simulink model "modelPredictiveControl_v0"  (R2024b)
settings: Solver=FixedStepAuto  StartTime=0.0  StopTime=80  FixedStep=0.01  RelTol=1e-3
undefined symbols (not defined in the file or in its folder): C, del_t, initial_conditions
libraries: mpclib x3
(part 1 of 2)
settings Model: Creator=sagar  LastModifiedBy=Sakar
settings RTWCC: GPUComputeCapability=3.5

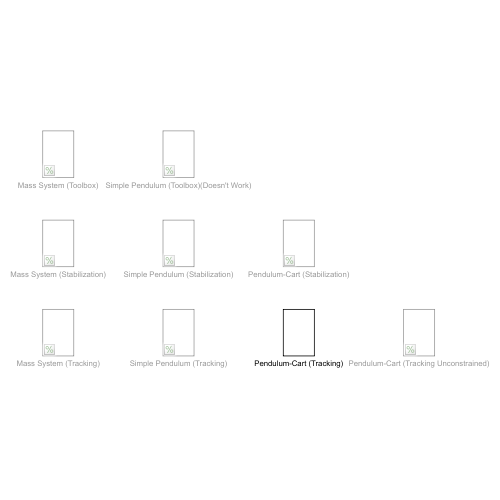
[thumbnail: Simulink's stored preview of the top-level diagram]
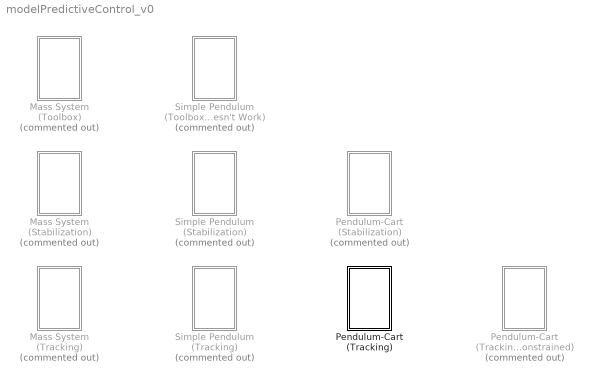
== system modelPredictiveControl_v0 ==
  Mass System (Stabilization) : Subsystem  Commented=on
  Mass System (Toolbox) : Subsystem  Commented=on
  Mass System (Tracking) : Subsystem  Commented=on
  Pendulum-Cart (Stabilization) : Subsystem  Commented=on
  Pendulum-Cart (Tracking Unconstrained) : Subsystem  Commented=on
  Pendulum-Cart (Tracking) : Subsystem
  Simple Pendulum (Stabilization) : Subsystem  Commented=on
  Simple Pendulum (Toolbox)(Doesn't Work) : Subsystem  Commented=on
  Simple Pendulum (Tracking) : Subsystem  Commented=on

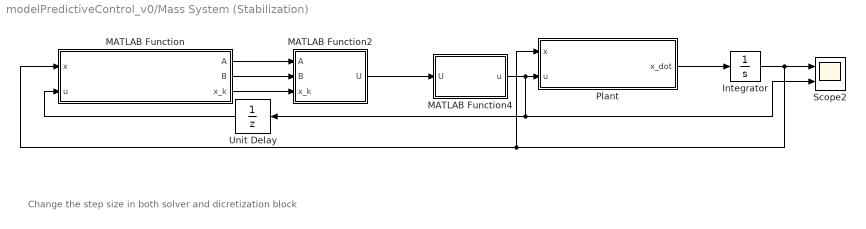
== system modelPredictiveControl_v0/Mass System (Stabilization) ==
  note: Change the step size in both solver and dicretization block
  Integrator : Integrator  InitialCondition=initial_conditions
  MATLAB Function : MATLAB Function  TreatAsAtomicUnit=on
  MATLAB Function2 : MATLAB Function  TreatAsAtomicUnit=on
  MATLAB Function4 : MATLAB Function  TreatAsAtomicUnit=on
  Plant : MATLAB Function  TreatAsAtomicUnit=on
  Scope2 : Scope  NumInputPorts=2
  Unit Delay : UnitDelay  SampleTime=-1  HasFrameUpgradeWarning=on
  wires:
  Plant/1(x_dot) -> Integrator/1
  Integrator/1 -> Scope2/1, Plant/1(x), MATLAB Function/1(x)
  MATLAB Function2/1(U) -> MATLAB Function4/1(U)
  MATLAB Function/1(A) -> MATLAB Function2/1(A)
  MATLAB Function/2(B) -> MATLAB Function2/2(B)
  MATLAB Function/3(x_k) -> MATLAB Function2/3(x_k)
  MATLAB Function4/1(u) -> Scope2/2, Unit Delay/1, Plant/2(u)
  Unit Delay/1 -> MATLAB Function/2(u)

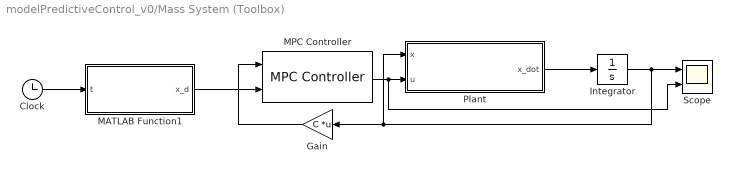
== system modelPredictiveControl_v0/Mass System (Toolbox) ==
  Clock : Clock
  Gain : Gain  Gain=C  Multiplication=Matrix(K*u)
  Integrator : Integrator  InitialCondition=initial_conditions
  MATLAB Function1 : MATLAB Function  TreatAsAtomicUnit=on
  MPC Controller : mpclib/MPC Controller  SCDEnableBlockLinearizationSpecification=on  mpcobj=mpc1  is_multiple=0  enable_value=0  return_u0=off  updateMPCinCallerWorkspace=on  md_inport=off  mv_inport=off  uref_inport=off  return_cost=off  return_mvseq=off  return_qpstatus=off  return_xseq=off  return_state=off  return_ovseq=off  state_inport=off  umin_inport=off  umax_inport=off  ymin_inport=off  ymax_inport=off  cc_inport=off  ywt_inport=off  uwt_inport=off  duwt_inport=off  rhoeps_inport=off  pm_inport=off  MaximumP=10  HorizonChoice=FixedHorizon  n_ts=0.01  n_p=50  n_mv=1  n_md=0  n_ud=0  n_mo=1  n_uo=0  BlockDataType=double  SampleTimeInherited=off  switch_inport=off
  Plant : MATLAB Function  TreatAsAtomicUnit=on
  Scope : Scope  NumInputPorts=2
  wires:
  MPC Controller/1 -> Scope/2, Plant/2(u)
  Plant/1(x_dot) -> Integrator/1
  Integrator/1 -> Scope/1, Plant/1(x), Gain/1
  Clock/1 -> MATLAB Function1/1(t)
  MATLAB Function1/1(x_d) -> MPC Controller/2
  Gain/1 -> MPC Controller/1

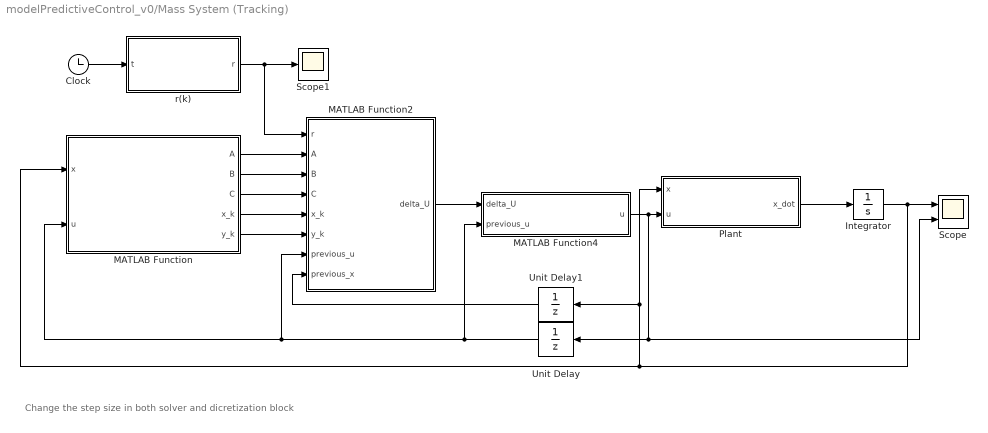
== system modelPredictiveControl_v0/Mass System (Tracking) ==
  note: Change the step size in both solver and dicretization block
  Clock : Clock
  Integrator : Integrator  InitialCondition=initial_conditions
  MATLAB Function : MATLAB Function  TreatAsAtomicUnit=on
  MATLAB Function2 : MATLAB Function  TreatAsAtomicUnit=on
  MATLAB Function4 : MATLAB Function  TreatAsAtomicUnit=on
  Plant : MATLAB Function  TreatAsAtomicUnit=on
  Scope : Scope  NumInputPorts=2
  Scope1 : Scope
  Unit Delay : UnitDelay  SampleTime=-1  HasFrameUpgradeWarning=on
  Unit Delay1 : UnitDelay  SampleTime=-1  HasFrameUpgradeWarning=on
  r(k) : MATLAB Function  TreatAsAtomicUnit=on
  wires:
  Plant/1(x_dot) -> Integrator/1
  Integrator/1 -> Scope/1, Unit Delay1/1, Plant/1(x), MATLAB Function/1(x)
  MATLAB Function2/1(delta_U) -> MATLAB Function4/1(delta_U)
  MATLAB Function/1(A) -> MATLAB Function2/2(A)
  MATLAB Function/2(B) -> MATLAB Function2/3(B)
  MATLAB Function/4(x_k) -> MATLAB Function2/5(x_k)
  MATLAB Function4/1(u) -> Unit Delay/1, Scope/2, Plant/2(u)
  Unit Delay/1 -> MATLAB Function4/2(previous_u), MATLAB Function/2(u), MATLAB Function2/7(previous_u)
  Clock/1 -> r(k)/1(t)
  r(k)/1(r) -> MATLAB Function2/1(r), Scope1/1
  MATLAB Function/3(C) -> MATLAB Function2/4(C)
  Unit Delay1/1 -> MATLAB Function2/8(previous_x)
  MATLAB Function/5(y_k) -> MATLAB Function2/6(y_k)

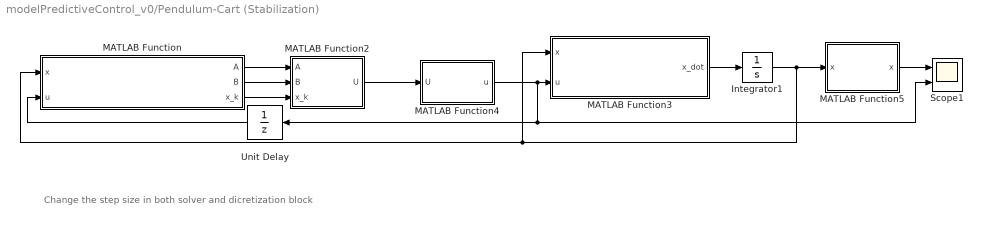
== system modelPredictiveControl_v0/Pendulum-Cart (Stabilization) ==
  note: Change the step size in both solver and dicretization block
  Integrator1 : Integrator  InitialCondition=initial_conditions
  MATLAB Function : MATLAB Function  TreatAsAtomicUnit=on
  MATLAB Function2 : MATLAB Function  TreatAsAtomicUnit=on
  MATLAB Function3 : MATLAB Function  TreatAsAtomicUnit=on
  MATLAB Function4 : MATLAB Function  TreatAsAtomicUnit=on
  MATLAB Function5 : MATLAB Function  TreatAsAtomicUnit=on
  Scope1 : Scope  NumInputPorts=2
  Unit Delay : UnitDelay  SampleTime=-1  HasFrameUpgradeWarning=on
  wires:
  MATLAB Function4/1(u) -> MATLAB Function3/2(u), Unit Delay/1, Scope1/2
  Unit Delay/1 -> MATLAB Function/2(u)
  MATLAB Function2/1(U) -> MATLAB Function4/1(U)
  MATLAB Function/3(x_k) -> MATLAB Function2/3(x_k)
  MATLAB Function/1(A) -> MATLAB Function2/1(A)
  Integrator1/1 -> MATLAB Function5/1("x "), MATLAB Function3/1(x), MATLAB Function/1(x)
  MATLAB Function/2(B) -> MATLAB Function2/2(B)
  MATLAB Function3/1(x_dot) -> Integrator1/1
  MATLAB Function5/1(x) -> Scope1/1

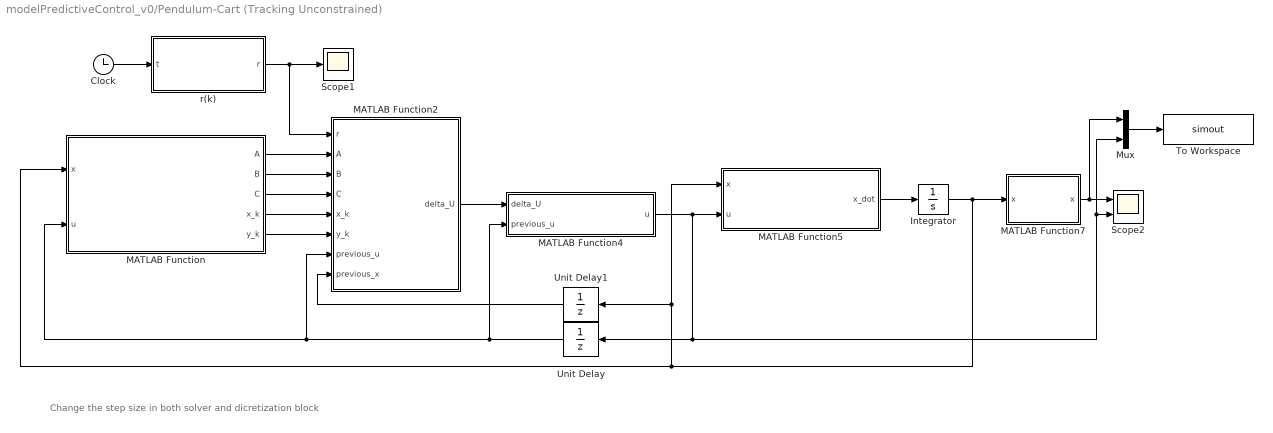
== system modelPredictiveControl_v0/Pendulum-Cart (Tracking Unconstrained) ==
  note: Change the step size in both solver and dicretization block
  Clock : Clock
  Integrator : Integrator  InitialCondition=initial_conditions
  MATLAB Function : MATLAB Function  TreatAsAtomicUnit=on
  MATLAB Function2 : MATLAB Function  TreatAsAtomicUnit=on
  MATLAB Function4 : MATLAB Function  TreatAsAtomicUnit=on
  MATLAB Function5 : MATLAB Function  TreatAsAtomicUnit=on
  MATLAB Function7 : MATLAB Function  TreatAsAtomicUnit=on
  Mux : Mux  Inputs=2
  Scope1 : Scope
  Scope2 : Scope  NumInputPorts=2
  To Workspace : ToWorkspace  VariableName=simout  SaveFormat=Timeseries  SampleTime=-1
  Unit Delay : UnitDelay  SampleTime=-1  HasFrameUpgradeWarning=on
  Unit Delay1 : UnitDelay  SampleTime=-1  HasFrameUpgradeWarning=on
  r(k) : MATLAB Function  TreatAsAtomicUnit=on
  wires:
  MATLAB Function5/1(x_dot) -> Integrator/1
  Integrator/1 -> MATLAB Function7/1("x "), MATLAB Function/1(x), MATLAB Function5/1(x), Unit Delay1/1
  MATLAB Function2/1(delta_U) -> MATLAB Function4/1(delta_U)
  MATLAB Function/1(A) -> MATLAB Function2/2(A)
  MATLAB Function/2(B) -> MATLAB Function2/3(B)
  MATLAB Function/4(x_k) -> MATLAB Function2/5(x_k)
  MATLAB Function4/1(u) -> MATLAB Function5/2(u), Mux/2, Scope2/2, Unit Delay/1
  Unit Delay/1 -> MATLAB Function4/2(previous_u), MATLAB Function/2(u), MATLAB Function2/7(previous_u)
  Clock/1 -> r(k)/1(t)
  r(k)/1(r) -> MATLAB Function2/1(r), Scope1/1
  MATLAB Function/3(C) -> MATLAB Function2/4(C)
  Unit Delay1/1 -> MATLAB Function2/8(previous_x)
  MATLAB Function/5(y_k) -> MATLAB Function2/6(y_k)
  MATLAB Function7/1(x) -> Mux/1, Scope2/1
  Mux/1 -> To Workspace/1

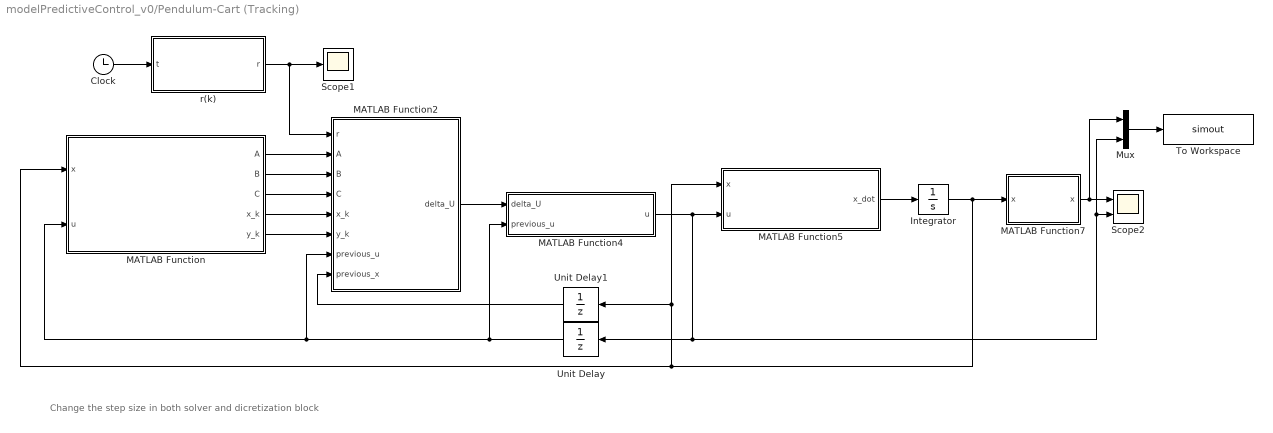
== system modelPredictiveControl_v0/Pendulum-Cart (Tracking) ==
  note: Change the step size in both solver and dicretization block
  Clock : Clock
  Integrator : Integrator  InitialCondition=initial_conditions
  MATLAB Function : MATLAB Function  TreatAsAtomicUnit=on
  MATLAB Function2 : MATLAB Function  TreatAsAtomicUnit=on
  MATLAB Function4 : MATLAB Function  TreatAsAtomicUnit=on
  MATLAB Function5 : MATLAB Function  TreatAsAtomicUnit=on
  MATLAB Function7 : MATLAB Function  TreatAsAtomicUnit=on
  Mux : Mux  Inputs=2
  Scope1 : Scope
  Scope2 : Scope  NumInputPorts=2
  To Workspace : ToWorkspace  VariableName=simout  SaveFormat=Timeseries  SampleTime=-1
  Unit Delay : UnitDelay  SampleTime=-1  HasFrameUpgradeWarning=on
  Unit Delay1 : UnitDelay  SampleTime=-1  HasFrameUpgradeWarning=on
  r(k) : MATLAB Function  TreatAsAtomicUnit=on
  wires:
  MATLAB Function5/1(x_dot) -> Integrator/1
  Integrator/1 -> MATLAB Function7/1("x "), MATLAB Function/1(x), MATLAB Function5/1(x), Unit Delay1/1
  MATLAB Function2/1(delta_U) -> MATLAB Function4/1(delta_U)
  MATLAB Function/1(A) -> MATLAB Function2/2(A)
  MATLAB Function/2(B) -> MATLAB Function2/3(B)
  MATLAB Function/4(x_k) -> MATLAB Function2/5(x_k)
  MATLAB Function4/1(u) -> MATLAB Function5/2(u), Mux/2, Scope2/2, Unit Delay/1
  Unit Delay/1 -> MATLAB Function4/2(previous_u), MATLAB Function/2(u), MATLAB Function2/7(previous_u)
  Clock/1 -> r(k)/1(t)
  r(k)/1(r) -> MATLAB Function2/1(r), Scope1/1
  MATLAB Function/3(C) -> MATLAB Function2/4(C)
  Unit Delay1/1 -> MATLAB Function2/8(previous_x)
  MATLAB Function/5(y_k) -> MATLAB Function2/6(y_k)
  MATLAB Function7/1(x) -> Mux/1, Scope2/1
  Mux/1 -> To Workspace/1

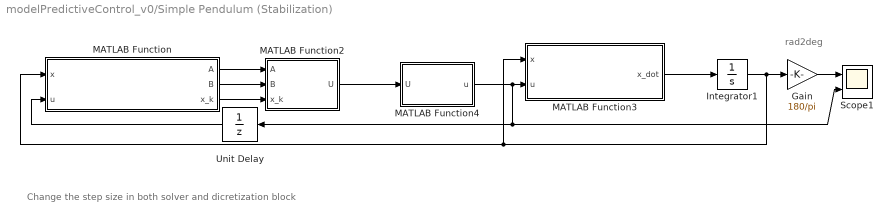
== system modelPredictiveControl_v0/Simple Pendulum (Stabilization) ==
  note: rad2deg
  note: Change the step size in both solver and dicretization block
  Gain : Gain  Gain=180/pi
  Integrator1 : Integrator  InitialCondition=initial_conditions
  MATLAB Function : MATLAB Function  TreatAsAtomicUnit=on
  MATLAB Function2 : MATLAB Function  TreatAsAtomicUnit=on
  MATLAB Function3 : MATLAB Function  TreatAsAtomicUnit=on
  MATLAB Function4 : MATLAB Function  TreatAsAtomicUnit=on
  Scope1 : Scope  NumInputPorts=2
  Unit Delay : UnitDelay  SampleTime=-1  HasFrameUpgradeWarning=on
  wires:
  MATLAB Function4/1(u) -> MATLAB Function3/2(u), Unit Delay/1, Scope1/2
  Unit Delay/1 -> MATLAB Function/2(u)
  MATLAB Function2/1(U) -> MATLAB Function4/1(U)
  MATLAB Function/3(x_k) -> MATLAB Function2/3(x_k)
  MATLAB Function/1(A) -> MATLAB Function2/1(A)
  Integrator1/1 -> Gain/1, MATLAB Function3/1(x), MATLAB Function/1(x)
  MATLAB Function/2(B) -> MATLAB Function2/2(B)
  MATLAB Function3/1(x_dot) -> Integrator1/1
  Gain/1 -> Scope1/1

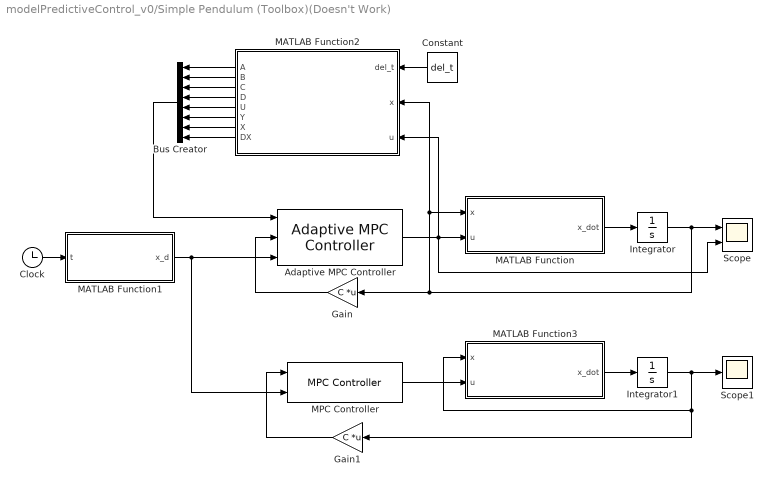
== system modelPredictiveControl_v0/Simple Pendulum (Toolbox)(Doesn't Work) ==
  Adaptive MPC Controller : mpclib/Adaptive MPC Controller  SCDEnableBlockLinearizationSpecification=on  mpcobj=mpc1  enable_value=0  updateMPCinCallerWorkspace=on  md_inport=off  mv_inport=off  uref_inport=off  return_cost=off  return_mvseq=off  return_qpstatus=off  return_xseq=off  return_state=off  return_ovseq=off  state_inport=off  isltv_plant=off  umin_inport=off  umax_inport=off  ymin_inport=off  ymax_inport=off  cc_inport=off  ywt_inport=off  uwt_inport=off  duwt_inport=off  rhoeps_inport=off  pm_inport=off  MaximumP=30  HorizonChoice=FixedHorizon  BlockDataType=double  SampleTimeInherited=off  switch_inport=off
  Bus Creator : BusCreator  Inputs=8
  Clock : Clock
  Constant : Constant  Value=del_t
  Gain : Gain  Gain=C  Multiplication=Matrix(K*u)
  Gain1 : Gain  Gain=C  Multiplication=Matrix(K*u)
  Integrator : Integrator  InitialCondition=initial_conditions
  Integrator1 : Integrator  InitialCondition=initial_conditions
  MATLAB Function : MATLAB Function  TreatAsAtomicUnit=on
  MATLAB Function1 : MATLAB Function  TreatAsAtomicUnit=on
  MATLAB Function2 : MATLAB Function  TreatAsAtomicUnit=on
  MATLAB Function3 : MATLAB Function  TreatAsAtomicUnit=on
  MPC Controller : mpclib/MPC Controller  SCDEnableBlockLinearizationSpecification=on  mpcobj=mpc1  is_multiple=0  enable_value=0  return_u0=off  updateMPCinCallerWorkspace=on  md_inport=off  mv_inport=off  uref_inport=off  return_cost=off  return_mvseq=off  return_qpstatus=off  return_xseq=off  return_state=off  return_ovseq=off  state_inport=off  umin_inport=off  umax_inport=off  ymin_inport=off  ymax_inport=off  cc_inport=off  ywt_inport=off  uwt_inport=off  duwt_inport=off  rhoeps_inport=off  pm_inport=off  MaximumP=10  HorizonChoice=FixedHorizon  n_ts=0.01  n_p=50  n_mv=1  n_md=0  n_ud=0  n_mo=1  n_uo=0  BlockDataType=double  SampleTimeInherited=off  switch_inport=off
  Scope : Scope  NumInputPorts=2
  Scope1 : Scope
  wires:
  Adaptive MPC Controller/1 -> MATLAB Function2/3(u), MATLAB Function/2(u), Scope/2
  MATLAB Function/1(x_dot) -> Integrator/1
  Integrator/1 -> Scope/1, MATLAB Function2/2(x), MATLAB Function/1(x), Gain/1
  Clock/1 -> MATLAB Function1/1(t)
  MATLAB Function1/1(x_d) -> Adaptive MPC Controller/3, MPC Controller/2
  Gain/1 -> Adaptive MPC Controller/2
  Constant/1 -> MATLAB Function2/1(del_t)
  Integrator1/1 -> Scope1/1, Gain1/1, MATLAB Function3/1(x)
  MPC Controller/1 -> MATLAB Function3/2(u)
  MATLAB Function3/1(x_dot) -> Integrator1/1
  Gain1/1 -> MPC Controller/1
  MATLAB Function2/1(A) -> Bus Creator/1
  MATLAB Function2/2(B) -> Bus Creator/2
  MATLAB Function2/3(C) -> Bus Creator/3
  MATLAB Function2/4(D) -> Bus Creator/4
  MATLAB Function2/5(U) -> Bus Creator/5
  MATLAB Function2/6(Y) -> Bus Creator/6
  MATLAB Function2/7(X) -> Bus Creator/7
  MATLAB Function2/8(DX) -> Bus Creator/8
  Bus Creator/1 -> Adaptive MPC Controller/1

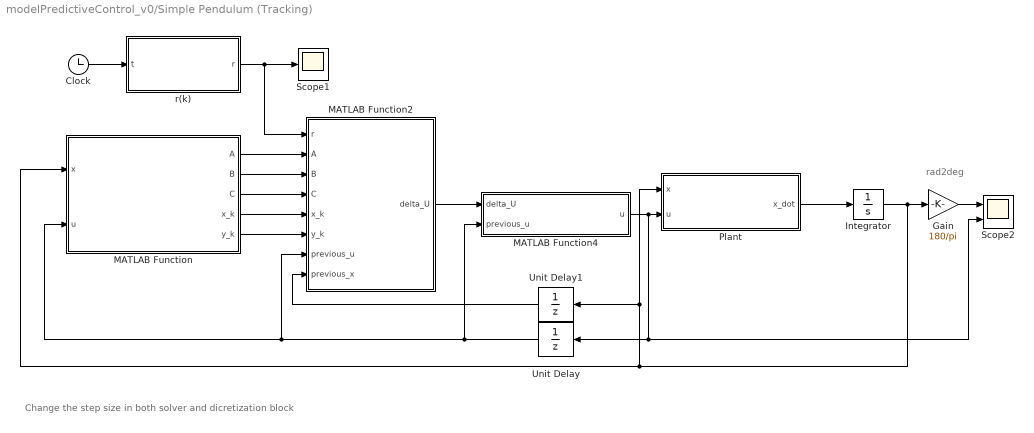
== system modelPredictiveControl_v0/Simple Pendulum (Tracking) ==
  note: Change the step size in both solver and dicretization block
  note: rad2deg
  Clock : Clock
  Gain : Gain  Gain=180/pi
  Integrator : Integrator  InitialCondition=initial_conditions
  MATLAB Function : MATLAB Function  TreatAsAtomicUnit=on
  MATLAB Function2 : MATLAB Function  TreatAsAtomicUnit=on
  MATLAB Function4 : MATLAB Function  TreatAsAtomicUnit=on
  Plant : MATLAB Function  TreatAsAtomicUnit=on
  Scope1 : Scope
  Scope2 : Scope  NumInputPorts=2
  Unit Delay : UnitDelay  SampleTime=-1  HasFrameUpgradeWarning=on
  Unit Delay1 : UnitDelay  SampleTime=-1  HasFrameUpgradeWarning=on
  r(k) : MATLAB Function  TreatAsAtomicUnit=on
  wires:
  Plant/1(x_dot) -> Integrator/1
  Integrator/1 -> Gain/1, Plant/1(x), Unit Delay1/1, MATLAB Function/1(x)
  MATLAB Function2/1(delta_U) -> MATLAB Function4/1(delta_U)
  MATLAB Function/1(A) -> MATLAB Function2/2(A)
  MATLAB Function/2(B) -> MATLAB Function2/3(B)
  MATLAB Function/4(x_k) -> MATLAB Function2/5(x_k)
  MATLAB Function4/1(u) -> Plant/2(u), Scope2/2, Unit Delay/1
  Unit Delay/1 -> MATLAB Function4/2(previous_u), MATLAB Function/2(u), MATLAB Function2/7(previous_u)
  Clock/1 -> r(k)/1(t)
  r(k)/1(r) -> MATLAB Function2/1(r), Scope1/1
  MATLAB Function/3(C) -> MATLAB Function2/4(C)
  Unit Delay1/1 -> MATLAB Function2/8(previous_x)
  MATLAB Function/5(y_k) -> MATLAB Function2/6(y_k)
  Gain/1 -> Scope2/1

== matlab function modelPredictiveControl_v0/Simple Pendulum (Toolbox)(Doesn't Work)/MATLAB Function3 ==
  data: x input; u input; x_dot output
function x_dot = pendulum_dynamics(x, u)
    g = 9.81; ell = 1;
    A = [0 1;
         -(g/ell) 0];
    B = [0; 1/ell];
    x_dot = A*x + B*u;
end

== matlab function modelPredictiveControl_v0/Mass System (Stabilization)/MATLAB Function ==
  data: x input; u input; A output; B output; x_k output
function [A, B, x_k] = discrete_mass_model(x, u)
    coder.extrinsic('ss');
    coder.extrinsic("c2d");
    coder.extrinsic("ssdata");
    % Continuous-time model
    Ac = [0 1;
          0 0];
    Bc = [0; 1];
    Cc = [1 0];
    Dc = [0];

    % % Discrete-time model Method 1
    % del_t = 0.01;
    % nx = size(Ac, 1);
    % nu = size(Bc, 2);
    % M = expm([[Ac Bc]*del_t; zeros(nu, nx+nu)]);
    % A = M(1:nx, 1:nx);
    % B = M(1:nx, nx+1:nx+nu);
    % C = Cc;
    % D = Dc;

    % Discrete-time model Method 2
    % Preinitializing the sizes of Ad, Bd, Cd, Dd
    A = Ac; B = Bc; C = Cc; D = Dc;
    % Discretization
    del_t = 0.01;
    [A, B, C, D] = ssdata(c2d(ss(Ac,Bc,Cc,Dc),del_t));
    x_k = x;
end

== matlab function modelPredictiveControl_v0/Mass System (Stabilization)/MATLAB Function2 ==
  data: A input; U output; B input; x_k input
function U = MPC(A, B, x_k)
    coder.extrinsic("quadprog");
    %% --------------------------------------------------------------------
    % Construct Ge = 2(upsilon + (gamma)' xi gamma)
    lx = 2;
    lu = 1;
    N = 30;   % MPC horizon
    
    % upsilon
    R = [.05];   % Cost weight for input
    R_array = repmat({R}, 1, N);
    upsilon = blkdiag(R_array{:});

    % xi
    Q = 1*eye(lx);    % Cost weight for state
    Q_array = repmat({Q}, 1, N-1);
    P = 1*eye(lx);
    xi = blkdiag(Q_array{:});
    xi = blkdiag(xi, P);

    % gamma
    gamma_first_col = zeros(N*lx, lu);
    % Create the first column of gamma, i.e., [B AB A^2B ... A^(N-1)B]'
    for i = 0:(N-1)
        j = A^i * B;
        gamma_first_col((i*lx + 1):((i+1)*lx), 1:lu) = j;
    end
    % Fill up the rest of the columns of gamma
    gamma = [gamma_first_col zeros(N*lx, N-1)];
    for i = 1:(N-1)
        j = gamma_first_col(1:(N-i)*lx, 1:lu);
        gamma((i*lx + 1):(N*lx), (i*lu + 1):((i+1)*lu)) = j;
    end

    % Ge
    Ge = 2 * (upsilon + transpose(gamma) * xi * gamma);
    %% --------------------------------------------------------------------

    %% --------------------------------------------------------------------
    % Construct F = 2 (gamma)' xi phi where phi = [A ... A^N]'

    % phi
    phi = zeros(N*lx, lx);
    for i = 1:N
        phi(((i-1)*lx + 1):i*lx, 1:lx) = A^i;
    end

    % F
    F = 2 * transpose(gamma) * xi * phi;
    %% --------------------------------------------------------------------

    %% --------------------------------------------------------------------
    % Construct J = eM gamma + epsilon

    % G (constraint on final state)
    G = [eye(lx);
         -eye(lx)];

    % eM
    M = [eye(lx);
         -eye(lx);
         zeros(lu, lx);
         zeros(lu, lx)];
    eM_upper_block = zeros(2*(lx + lu), N*lx);
    M_array = repmat({M}, 1, N-1);
    eM_lower_block = blkdiag(M_array{:});
    eM_lower_block = blkdiag(eM_lower_block, G);
    eM = [eM_upper_block; eM_lower_block];

    % epsilon
    E = [zeros(lx, lu);
         zeros(lx, lu);
         eye(lu);
         -eye(lu)];
    E_array = repmat({E}, 1, N);
    epsilon_upper_block = blkdiag(E_array{:});
    epsilon_lower_block = zeros(2*lx, N*lu);
    epsilon = [epsilon_upper_block; epsilon_lower_block];

    % J
    J = eM * gamma + epsilon;
    %% --------------------------------------------------------------------

    %% --------------------------------------------------------------------
    % Construct c = [f_0 f_1 ... f_(N-1) h]'

    % f
    f_u = [80;
           80];   % Constraints on input
    f_x = [11;
           30;
           11;
           30];    % Constraints on state
    h = [11;
         30;
         11;
         30];      % Constraints on the final state

    f = [f_x; f_u];

    % c
    c = kron(ones(N, 1), f);
    c = [c; h];
    %% --------------------------------------------------------------------

    %% --------------------------------------------------------------------
    % Construct Wo = -eM phi - De where De = [M_0 0 0 ... 0]'

    % De
    M_0 = [eye(lx);
           -eye(lx);
           zeros(lu, lx);
           zeros(lu, lx)];
    De_lower_block = zeros(2*N*(lx+lu) - 2*lu, lx);
    De = [M_0; De_lower_block];

    % Wo
    Wo = -eM * phi - De;
    %% --------------------------------------------------------------------

    %% --------------------------------------------------------------------
    % Setting up quadprog
    b = c + Wo * x_k;
    f = F * x_k;
    U = zeros(N*lu, 1);
    U = quadprog(Ge,f,J,b);
    %% --------------------------------------------------------------------

end

== matlab function modelPredictiveControl_v0/Pendulum-Cart (Tracking Unconstrained)/MATLAB Function4 ==
  data: delta_U input; u output; previous_u input
function u = first_u(delta_U, previous_u)
    lu = 1;
    u = previous_u + delta_U(1:lu);
end

== matlab function modelPredictiveControl_v0/Mass System (Stabilization)/MATLAB Function4 ==
  data: U input; u output
function u = first_u(U)
    lu = 1;
    u = U(1:lu);
end

== matlab function modelPredictiveControl_v0/Simple Pendulum (Stabilization)/MATLAB Function ==
  data: x input; u input; A output; B output; x_k output
function [A, B, x_k] = discrete_pendulum_model(x, u)
    coder.extrinsic('ss');
    coder.extrinsic("c2d");
    coder.extrinsic("ssdata");
    % Physical Parameters
    g = 9.81; ell = 1;

    % Continuous-time model
    Ac = [0 1;
          -(g/ell) * cos(x(1)) 0];
    Bc = [0; 1/ell];
    Cc = [1 0];
    Dc = [0];

    % % Discrete-time model Method 1
    % del_t = 0.01;
    % nx = size(Ac, 1);
    % nu = size(Bc, 2);
    % M = expm([[Ac Bc]*del_t; zeros(nu, nx+nu)]);
    % A = M(1:nx, 1:nx);
    % B = M(1:nx, nx+1:nx+nu);
    % C = Cc;
    % D = Dc;

    % Discrete-time model Method 2
    % Preinitializing the sizes of Ad, Bd, Cd, Dd
    A = Ac; B = Bc; C = Cc; D = Dc;
    % Discretization
    del_t = 0.01;
    [A, B, C, D] = ssdata(c2d(ss(Ac,Bc,Cc,Dc),del_t));
    x_k = x;
end

== matlab function modelPredictiveControl_v0/Simple Pendulum (Stabilization)/MATLAB Function2 ==
  data: A input; U output; B input; x_k input
function U = MPC(A, B, x_k)
    coder.extrinsic("quadprog");
    %% --------------------------------------------------------------------
    % Construct Ge = 2(upsilon + (gamma)' xi gamma)
    lx = 2;
    lu = 1;
    N = 30;   % MPC horizon
    
    % upsilon
    R = [.05];   % Cost weight for input
    R_array = repmat({R}, 1, N);
    upsilon = blkdiag(R_array{:});

    % xi
    Q = 1*eye(lx);    % Cost weight for state
    Q_array = repmat({Q}, 1, N-1);
    P = 1*eye(lx);
    xi = blkdiag(Q_array{:});
    xi = blkdiag(xi, P);

    % gamma
    gamma_first_col = zeros(N*lx, lu);
    % Create the first column of gamma, i.e., [B AB A^2B ... A^(N-1)B]'
    for i = 0:(N-1)
        j = A^i * B;
        gamma_first_col((i*lx + 1):((i+1)*lx), 1:lu) = j;
    end
    % Fill up the rest of the columns of gamma
    gamma = [gamma_first_col zeros(N*lx, N-1)];
    for i = 1:(N-1)
        j = gamma_first_col(1:(N-i)*lx, 1:lu);
        gamma((i*lx + 1):(N*lx), (i*lu + 1):((i+1)*lu)) = j;
    end

    % Ge
    Ge = 2 * (upsilon + transpose(gamma) * xi * gamma);
    %% --------------------------------------------------------------------

    %% --------------------------------------------------------------------
    % Construct F = 2 (gamma)' xi phi where phi = [A ... A^N]'

    % phi
    phi = zeros(N*lx, lx);
    for i = 1:N
        phi(((i-1)*lx + 1):i*lx, 1:lx) = A^i;
    end

    % F
    F = 2 * transpose(gamma) * xi * phi;
    %% --------------------------------------------------------------------

    %% --------------------------------------------------------------------
    % Construct J = eM gamma + epsilon

    % G (constraint on final state)
    G = [eye(lx);
         -eye(lx)];

    % eM
    M = [eye(lx);
         -eye(lx);
         zeros(lu, lx);
         zeros(lu, lx)];
    eM_upper_block = zeros(2*(lx + lu), N*lx);
    M_array = repmat({M}, 1, N-1);
    eM_lower_block = blkdiag(M_array{:});
    eM_lower_block = blkdiag(eM_lower_block, G);
    eM = [eM_upper_block; eM_lower_block];

    % epsilon
    E = [zeros(lx, lu);
         zeros(lx, lu);
         eye(lu);
         -eye(lu)];
    E_array = repmat({E}, 1, N);
    epsilon_upper_block = blkdiag(E_array{:});
    epsilon_lower_block = zeros(2*lx, N*lu);
    epsilon = [epsilon_upper_block; epsilon_lower_block];

    % J
    J = eM * gamma + epsilon;
    %% --------------------------------------------------------------------

    %% --------------------------------------------------------------------
    % Construct c = [f_0 f_1 ... f_(N-1) h]'

    % f
    f_u = [80;
           80];   % Constraints on input
    f_x = [10;
           30;
           10;
           30];    % Constraints on state
    h = [10;
         30;
         10;
         30];      % Constraints on the final state

    f = [f_x; f_u];

    % c
    c = kron(ones(N, 1), f);
    c = [c; h];
    %% --------------------------------------------------------------------

    %% --------------------------------------------------------------------
    % Construct Wo = -eM phi - De where De = [M_0 0 0 ... 0]'

    % De
    M_0 = [eye(lx);
           -eye(lx);
           zeros(lu, lx);
           zeros(lu, lx)];
    De_lower_block = zeros(2*N*(lx+lu) - 2*lu, lx);
    De = [M_0; De_lower_block];

    % Wo
    Wo = -eM * phi - De;
    %% --------------------------------------------------------------------

    %% --------------------------------------------------------------------
    % Setting up quadprog
    b = c + Wo * x_k;
    f = F * x_k;
    U = zeros(N*lu, 1);
    U = quadprog(Ge,f,J,b);
    %% --------------------------------------------------------------------

end

== matlab function modelPredictiveControl_v0/Simple Pendulum (Stabilization)/MATLAB Function4 ==
  data: U input; u output
function u = first_u(U)
    lu = 1;
    u = U(1:lu);
end

== matlab function modelPredictiveControl_v0/Simple Pendulum (Stabilization)/MATLAB Function3 ==
  data: x input; u input; x_dot output
function x_dot = pendulum_dynamics(x, u)
    g = 9.81; l = 1;
    x_dot = [x(2);
             -(g/l) * sin(x(1)) + (1/l) * u];
end

== matlab function modelPredictiveControl_v0/Pendulum-Cart (Tracking Unconstrained)/MATLAB Function5 ==
  data: x input; u input; x_dot output
function x_dot = pendulum_cart_dynamics(x, u)
    m1 = 1; m2 = 1; l = 0.1; k = 0; g = 9.81; kappa = 0;

    f_x_1 = x(2);
    f_x_2 = 1/(m1 + m2 - m2 * (cos(x(3)))^2) * ...
             (m2 * g * sin(x(3)) * cos(x(3)) + (kappa/l) * cos(x(3)) * x(3) + ...
             k * x(1) + m2 * l * sin(x(3)) * x(4)^2);
    f_x_3 = x(4);
    f_x_4 = f_x_2 * (-cos(x(3))/l) - (g/l) * sin(x(3)) - ...
             (kappa/(m2*l^2)) * x(3);
    f_x = [f_x_1; f_x_2; f_x_3; f_x_4];
    
    g_x = [0;
           1/(m1 + m2 - m2 * cos(x(3))^2);
           0;
           (-cos(x(3))/l) * (1/(m1 + m2 - m2 * cos(x(3))^2))];

    x_dot = f_x + g_x * u;
end

== matlab function modelPredictiveControl_v0/Pendulum-Cart (Stabilization)/MATLAB Function2 ==
  data: A input; U output; B input; x_k input
function U = MPC(A, B, x_k)
    coder.extrinsic("quadprog");
    %% --------------------------------------------------------------------
    % Construct Ge = 2(upsilon + (gamma)' xi gamma)
    lx = 4;
    lu = 1;
    N = 30;   % MPC horizon
    
    % upsilon
    R = [0.1];   % Cost weight for input
    R_array = repmat({R}, 1, N);
    upsilon = blkdiag(R_array{:});

    % xi
    Q = 10*eye(lx);    % Cost weight for state
    Q_array = repmat({Q}, 1, N-1);
    P = 10*eye(lx);
    xi = blkdiag(Q_array{:});
    xi = blkdiag(xi, P);

    % gamma
    gamma_first_col = zeros(N*lx, lu);
    % Create the first column of gamma, i.e., [B AB A^2B ... A^(N-1)B]'
    for i = 0:(N-1)
        j = A^i * B;
        gamma_first_col((i*lx + 1):((i+1)*lx), 1:lu) = j;
    end
    % Fill up the rest of the columns of gamma
    gamma = [gamma_first_col zeros(N*lx, N-1)];
    for i = 1:(N-1)
        j = gamma_first_col(1:(N-i)*lx, 1:lu);
        gamma((i*lx + 1):(N*lx), (i*lu + 1):((i+1)*lu)) = j;
    end

    % Ge
    Ge = 2 * (upsilon + transpose(gamma) * xi * gamma);
    %% --------------------------------------------------------------------

    %% --------------------------------------------------------------------
    % Construct F = 2 (gamma)' xi phi where phi = [A ... A^N]'

    % phi
    phi = zeros(N*lx, lx);
    for i = 1:N
        phi(((i-1)*lx + 1):i*lx, 1:lx) = A^i;
    end

    % F
    F = 2 * transpose(gamma) * xi * phi;
    %% --------------------------------------------------------------------

    %% --------------------------------------------------------------------
    % Construct J = eM gamma + epsilon

    % G (constraint on final state)
    G = [eye(lx);
         -eye(lx)];

    % eM
    M = [eye(lx);
         -eye(lx);
         zeros(lu, lx);
         zeros(lu, lx)];
    eM_upper_block = zeros(2*(lx + lu), N*lx);
    M_array = repmat({M}, 1, N-1);
    eM_lower_block = blkdiag(M_array{:});
    eM_lower_block = blkdiag(eM_lower_block, G);
    eM = [eM_upper_block; eM_lower_block];

    % epsilon
    E = [zeros(lx, lu);
         zeros(lx, lu);
         eye(lu);
         -eye(lu)];
    E_array = repmat({E}, 1, N);
    epsilon_upper_block = blkdiag(E_array{:});
    epsilon_lower_block = zeros(2*lx, N*lu);
    epsilon = [epsilon_upper_block; epsilon_lower_block];

    % J
    J = eM * gamma + epsilon;
    %% --------------------------------------------------------------------

    %% --------------------------------------------------------------------
    % Construct c = [f_0 f_1 ... f_(N-1) h]'

    % f
    f_u = [80;
           80];   % Constraints on input
    f_x = [10;
           10;
           10;
           20;
           10;
           10;
           10;
           20];    % Constraints on state
    h = [10;
         10;
         10;
         20;
         10;
         10;
         10;
         20];      % Constraints on the final state

    f = [f_x; f_u];

    % c
    c = kron(ones(N, 1), f);
    c = [c; h];
    %% --------------------------------------------------------------------

    %% --------------------------------------------------------------------
    % Construct Wo = -eM phi - De where De = [M_0 0 0 ... 0]'

    % De
    M_0 = [eye(lx);
           -eye(lx);
           zeros(lu, lx);
           zeros(lu, lx)];
    De_lower_block = zeros(2*N*(lx+lu) - 2*lu, lx);
    De = [M_0; De_lower_block];

    % Wo
    Wo = -eM * phi - De;
    %% --------------------------------------------------------------------

    %% --------------------------------------------------------------------
    % Setting up quadprog
    b = c + Wo * x_k;
    f = F * x_k;
    U = zeros(N*lu, 1);
    U = quadprog(Ge,f,J,b);
    %% --------------------------------------------------------------------

end

== matlab function modelPredictiveControl_v0/Mass System (Toolbox)/MATLAB Function1 ==
  data: t input; x_d output
function x_d = desired_trajectory(t)
    x_d = -5;
    if t < 2
        x_d = 2;
    end
end

== matlab function modelPredictiveControl_v0/Pendulum-Cart (Stabilization)/MATLAB Function3 ==
  data: x input; u input; x_dot output
function x_dot = pendulum_cart_dynamics(x, u)
    m1 = 1; m2 = 1; l = 0.1; k = 0; g = 9.81; kappa = 0;

    f_x_1 = x(2);
    f_x_2 = 1/(m1 + m2 - m2 * (cos(x(3)))^2) * ...
             (m2 * g * sin(x(3)) * cos(x(3)) + (kappa/l) * cos(x(3)) * x(3) + ...
             k * x(1) + m2 * l * sin(x(3)) * x(4)^2);
    f_x_3 = x(4);
    f_x_4 = f_x_2 * (-cos(x(3))/l) - (g/l) * sin(x(3)) - ...
             (kappa/(m2*l^2)) * x(3);
    f_x = [f_x_1; f_x_2; f_x_3; f_x_4];
    
    g_x = [0;
           1/(m1 + m2 - m2 * cos(x(3))^2);
           0;
           (-cos(x(3))/l) * (1/(m1 + m2 - m2 * cos(x(3))^2))];

    x_dot = f_x + g_x * u;
end

== matlab function modelPredictiveControl_v0/Pendulum-Cart (Stabilization)/MATLAB Function4 ==
  data: U input; u output
function u = first_u(U)
    lu = 1;
    u = U(1:lu);
    % u = 0;
end

== matlab function modelPredictiveControl_v0/Pendulum-Cart (Stabilization)/MATLAB Function5 ==
  data: x input; x output
function x = rad_to_deg(x)
    x(3) = rad2deg(x(3));
    x(4) = rad2deg(x(4));
end

== matlab function modelPredictiveControl_v0/Mass System (Tracking)/MATLAB Function ==
  data: x input; u input; A output; B output; C output; x_k output; y_k output
function [A, B, C, x_k, y_k] = discrete_mass_model(x, u)
    coder.extrinsic('ss');
    coder.extrinsic("c2d");
    coder.extrinsic("ssdata");
    % Continuous-time model
    Ac = [0 1;
          0 0];
    Bc = [0; 1];
    Cc = [1 0];
    Dc = [0];

    % % Discrete-time model Method 1
    % del_t = 0.01;
    % nx = size(Ac, 1);
    % nu = size(Bc, 2);
    % M = expm([[Ac Bc]*del_t; zeros(nu, nx+nu)]);
    % A = M(1:nx, 1:nx);
    % B = M(1:nx, nx+1:nx+nu);
    % C = Cc;
    % D = Dc;

    % Discrete-time model Method 2
    % Preinitializing the sizes of Ad, Bd, Cd, Dd
    A = Ac; B = Bc; C = Cc; D = Dc;
    % Discretization
    del_t = 0.01;
    [A, B, C, D] = ssdata(c2d(ss(Ac,Bc,Cc,Dc),del_t));
    x_k = x;
    y_k = C*x_k;
end

== matlab function modelPredictiveControl_v0/Mass System (Tracking)/r(k) ==
  data: t input; r output
function r = reference_trajectory(t)
    N_x = 30;
    set_point = [5];
    r = kron(ones(N_x, 1), set_point);
end

== matlab function modelPredictiveControl_v0/Mass System (Tracking)/MATLAB Function2 ==
  data: r input; A input; delta_U output; B input; C input; x_k input; y_k input; previous_u input; previous_x input
function delta_U = MPC(r, A, B, C, x_k, y_k, previous_u, previous_x)
    coder.extrinsic("quadprog");
    lx = 2;
    ly = 1;
    lu = 1;
    Nx = 30;    % Prediction horizon
    Nu = 5;     % Control horizon

    %% --------------------------------------------------------------------
    % Construct Ge = 2(upsilon + (gamma)' xi gamma)    
    % upsilon
    R = 0.05*eye(lu);   % Cost weight for change in input (delta u)
    upsilon = kron(eye(Nu), R);

    % xi
    Q = 1*eye(ly);    % Cost weight for state
    P = 1*eye(ly);
    xi = kron(eye(Nx-1), Q);
    xi = blkdiag(xi, P);

    % gamma
    Ce = [zeros(ly,lx) eye(ly)];
    Be = zeros(lx+ly, lu);
    % Be(1:lx, 1:lu) = B;
    % Be((lx+1):(lx+ly), 1:lu) = C*B;
    Be = [B; C*B];
    Ae = zeros(lx+ly);
    Ae(1:lx, 1:lx) = A;
    Ae((lx + 1):(lx + ly), 1:lx) = C*A;
    Ae((lx + 1):(lx + ly), (lx + 1):(lx + ly)) = eye(ly);

    gamma_first_col = zeros(Nx*ly, lu);
    % Create the first column of gamma, i.e., [CeBe CeAeBe ... CeAe^(Nx-1)Be]'
    for i = 0:(Nx-1)
        j = Ce * Ae^i * Be;
        gamma_first_col((i*ly + 1):((i+1)*ly), 1:lu) = j;
    end
    % Fill up rest of the gamma
    gamma = [gamma_first_col zeros(Nx*ly, (Nu-1)*lu)];
    for i = 1:(Nu-1)
        j = gamma_first_col(1:(Nx-i)*ly, 1:lu);
        gamma((i*ly + 1):(Nx*ly), (i*lu + 1):((i+1)*lu)) = j;
    end

    % Ge
    Ge = 2 * (upsilon + transpose(gamma) * xi * gamma);
    %% --------------------------------------------------------------------

    %% --------------------------------------------------------------------
    % Construct X = [delta_x  y]', Te = [X  previous_u  r]'
    
    % X
    delta_x = x_k - previous_x;
    X = [delta_x;
         y_k];

    % Te
    Te = [X;
          previous_u;
          r];
    %% --------------------------------------------------------------------

    %% --------------------------------------------------------------------
    % Construct eF = [2 (phi)' xi gamma    0    -2 xi gamma]'
    % where phi = [CeAe ... CeAe^(Nx)]'

    % phi
    phi = zeros(Nx*ly, (lx + ly));
    for i = 1:Nx
        phi(((i-1)*ly + 1):i*ly, 1:(lx + ly)) = Ce*Ae^i;
    end

    % eF
    eF = [2 * transpose(phi) * xi * gamma;
          zeros(lu, Nu*lu);
         -2 * xi * gamma];
    %% --------------------------------------------------------------------

    %% --------------------------------------------------------------------
    % Construct J = [-L  L  -I  I  gamma  -gamma]'

    % L
    lower_triangluar_ones = tril(ones(Nu));
    L = kron(lower_triangluar_ones, eye(lu));

    % J
    J = [-L;
          L;
         -eye(Nu*lu);
          eye(Nu*lu);
          gamma;
         -gamma];
    %% --------------------------------------------------------------------

    %% --------------------------------------------------------------------
    % Construct Wo = [-u0_min ... -u(Nu-1)_min  u0_max ... u(Nu-1)_max
    %                 -delta_u0_min ... -delta_u(Nu-1)_min  delta_u0_max ... delta_u(Nu-1)_max
    %                 -e1_min ... -e(Nx)_min  e1_max ... e(Nx)_max]'

    % Constraints on u
    u_min = [-800];
    u_max = [800];
    Wo_upper_block = [kron(-ones(Nu,1), u_min); kron(ones(Nu,1), u_max)];

    % Constraints on delta u
    delta_u_min = [-800];
    delta_u_max = [800];
    Wo_middle_block = [kron(-ones(Nu,1), delta_u_min); kron(ones(Nu,1), delta_u_max)];

    % Constraints on tracking error
    e_min = [-500];
    e_max = [500];
    Wo_lower_block = [kron(-ones(Nx,1), e_min); kron(ones(Nx,1), e_max)];

    Wo = [Wo_upper_block; Wo_middle_block; Wo_lower_block];
    %% --------------------------------------------------------------------

    %% --------------------------------------------------------------------
    % Construct eX
    
    % iota
    iota = kron(ones(Nu,1), eye(lu));

    % eX
    eX = [zeros(Nu*lu, lx+ly), iota, zeros(Nu*lu, Nx*ly);
          zeros(Nu*lu, lx+ly), -iota, zeros(Nu*lu, Nx*ly);
          zeros(2*Nu*lu, lx+ly + lu + Nx*ly);
          -phi, zeros(Nx*ly, lu), -eye(Nx*ly);
          phi, zeros(Nx*ly, lu), eye(Nx*ly)];
    %% --------------------------------------------------------------------

    %% --------------------------------------------------------------------
    % Setting up quadprog
    b = Wo + eX * Te;
    f = transpose(Te) * eF;
    delta_U = zeros(Nu*lu, 1);
    delta_U = quadprog(Ge,f,J,b);
    %% --------------------------------------------------------------------

end

== matlab function modelPredictiveControl_v0/Simple Pendulum (Tracking)/MATLAB Function ==
  data: x input; u input; A output; B output; C output; x_k output; y_k output
function [A, B, C, x_k, y_k] = discrete_pendulum_model(x, u)
    coder.extrinsic('ss');
    coder.extrinsic("c2d");
    coder.extrinsic("ssdata");
    % Physical Parameters
    g = 9.81; ell = 1;

    % Continuous-time model
    Ac = [0 1;
          -(g/ell) * cos(x(1)) 0];
    Bc = [0; 1/ell];
    Cc = [1 0];
    Dc = [0];

    % % Discrete-time model Method 1
    % del_t = 0.01;
    % nx = size(Ac, 1);
    % nu = size(Bc, 2);
    % M = expm([[Ac Bc]*del_t; zeros(nu, nx+nu)]);
    % A = M(1:nx, 1:nx);
    % B = M(1:nx, nx+1:nx+nu);
    % C = Cc;
    % D = Dc;

    % Discrete-time model Method 2
    % Preinitializing the sizes of Ad, Bd, Cd, Dd
    A = Ac; B = Bc; C = Cc; D = Dc;
    % Discretization
    del_t = 0.01;
    [A, B, C, D] = ssdata(c2d(ss(Ac,Bc,Cc,Dc),del_t));
    x_k = x;
    y_k = C*x_k;
end

== matlab function modelPredictiveControl_v0/Mass System (Toolbox)/Plant ==
  data: x input; u input; x_dot output
function x_dot = simple_mass_system(x, u)
    A = [0 1; 0 0];
    B = [0; 1];

    x_dot = A*x + B.*u;
end

== matlab function modelPredictiveControl_v0/Mass System (Tracking)/MATLAB Function4 ==
  data: delta_U input; u output; previous_u input
function u = first_u(delta_U, previous_u)
    lu = 1;
    u = previous_u + delta_U(1:lu);
end

== matlab function modelPredictiveControl_v0/Mass System (Tracking)/Plant ==
  data: x input; u input; x_dot output
function x_dot = simple_mass_system(x, u)
    A = [0 1; 0 0];
    B = [0; 1];

    x_dot = A*x + B.*u;
end

== matlab function modelPredictiveControl_v0/Simple Pendulum (Tracking)/MATLAB Function2 ==
  data: r input; A input; delta_U output; B input; C input; x_k input; y_k input; previous_u input; previous_x input
function delta_U = MPC(r, A, B, C, x_k, y_k, previous_u, previous_x)
    coder.extrinsic("quadprog");
    lx = 2;
    ly = 1;
    lu = 1;
    Nx = 30;    % Prediction horizon
    Nu = 5;     % Control horizon

    %% --------------------------------------------------------------------
    % Construct Ge = 2(upsilon + (gamma)' xi gamma)    
    % upsilon
    R = 0.05*eye(lu);   % Cost weight for change in input (delta u)
    upsilon = kron(eye(Nu), R);

    % xi
    Q = 1*eye(ly);    % Cost weight for state
    P = 1*eye(ly);
    xi = kron(eye(Nx-1), Q);
    xi = blkdiag(xi, P);

    % gamma
    Ce = [zeros(ly,lx) eye(ly)];
    Be = zeros(lx+ly, lu);
    % Be(1:lx, 1:lu) = B;
    % Be((lx+1):(lx+ly), 1:lu) = C*B;
    Be = [B; C*B];
    Ae = zeros(lx+ly);
    Ae(1:lx, 1:lx) = A;
    Ae((lx + 1):(lx + ly), 1:lx) = C*A;
    Ae((lx + 1):(lx + ly), (lx + 1):(lx + ly)) = eye(ly);

    gamma_first_col = zeros(Nx*ly, lu);
    % Create the first column of gamma, i.e., [CeBe CeAeBe ... CeAe^(Nx-1)Be]'
    for i = 0:(Nx-1)
        j = Ce * Ae^i * Be;
        gamma_first_col((i*ly + 1):((i+1)*ly), 1:lu) = j;
    end
    % Fill up rest of the gamma
    gamma = [gamma_first_col zeros(Nx*ly, (Nu-1)*lu)];
    for i = 1:(Nu-1)
        j = gamma_first_col(1:(Nx-i)*ly, 1:lu);
        gamma((i*ly + 1):(Nx*ly), (i*lu + 1):((i+1)*lu)) = j;
    end

    % Ge
    Ge = 2 * (upsilon + transpose(gamma) * xi * gamma);
    %% --------------------------------------------------------------------

    %% --------------------------------------------------------------------
    % Construct X = [delta_x  y]', Te = [X  previous_u  r]'
    
    % X
    delta_x = x_k - previous_x;
    X = [delta_x;
         y_k];

    % Te
    Te = [X;
          previous_u;
          r];
    %% --------------------------------------------------------------------

    %% --------------------------------------------------------------------
    % Construct eF = [2 (phi)' xi gamma    0    -2 xi gamma]'
    % where phi = [CeAe ... CeAe^(Nx)]'

    % phi
    phi = zeros(Nx*ly, (lx + ly));
    for i = 1:Nx
        phi(((i-1)*ly + 1):i*ly, 1:(lx + ly)) = Ce*Ae^i;
    end

    % eF
    eF = [2 * transpose(phi) * xi * gamma;
          zeros(lu, Nu*lu);
         -2 * xi * gamma];
    %% --------------------------------------------------------------------

    %% --------------------------------------------------------------------
    % Construct J = [-L  L  -I  I  gamma  -gamma]'

    % L
    lower_triangluar_ones = tril(ones(Nu));
    L = kron(lower_triangluar_ones, eye(lu));

    % J
    J = [-L;
          L;
         -eye(Nu*lu);
          eye(Nu*lu);
          gamma;
         -gamma];
    %% --------------------------------------------------------------------

    %% --------------------------------------------------------------------
    % Construct Wo = [-u0_min ... -u(Nu-1)_min  u0_max ... u(Nu-1)_max
    %                 -delta_u0_min ... -delta_u(Nu-1)_min  delta_u0_max ... delta_u(Nu-1)_max
    %                 -e1_min ... -e(Nx)_min  e1_max ... e(Nx)_max]'

    % Constraints on u
    u_min = [-200];
    u_max = [200];
    Wo_upper_block = [kron(-ones(Nu,1), u_min); kron(ones(Nu,1), u_max)];

    % Constraints on delta u
    delta_u_min = [-800];
    delta_u_max = [800];
    Wo_middle_block = [kron(-ones(Nu,1), delta_u_min); kron(ones(Nu,1), delta_u_max)];

    % Constraints on tracking error
    e_min = [-500];
    e_max = [500];
    Wo_lower_block = [kron(-ones(Nx,1), e_min); kron(ones(Nx,1), e_max)];

    Wo = [Wo_upper_block; Wo_middle_block; Wo_lower_block];
    %% --------------------------------------------------------------------

    %% --------------------------------------------------------------------
    % Construct eX
    
    % iota
    iota = kron(ones(Nu,1), eye(lu));

    % eX
    eX = [zeros(Nu*lu, lx+ly), iota, zeros(Nu*lu, Nx*ly);
          zeros(Nu*lu, lx+ly), -iota, zeros(Nu*lu, Nx*ly);
          zeros(2*Nu*lu, lx+ly + lu + Nx*ly);
          -phi, zeros(Nx*ly, lu), -eye(Nx*ly);
          phi, zeros(Nx*ly, lu), eye(Nx*ly)];
    %% --------------------------------------------------------------------

    %% --------------------------------------------------------------------
    % Setting up quadprog
    b = Wo + eX * Te;
    f = transpose(Te) * eF;
    delta_U = zeros(Nu*lu, 1);
    delta_U = quadprog(Ge,f,J,b);
    %% --------------------------------------------------------------------

end

== matlab function modelPredictiveControl_v0/Simple Pendulum (Tracking)/MATLAB Function4 ==
  data: delta_U input; u output; previous_u input
function u = first_u(delta_U, previous_u)
    lu = 1;
    u = previous_u + delta_U(1:lu);
end

== matlab function modelPredictiveControl_v0/Pendulum-Cart (Tracking Unconstrained)/MATLAB Function7 ==
  data: x input; x output
function x = rad_to_deg(x)
    x(3) = rad2deg(x(3));
    x(4) = rad2deg(x(4));
end

== matlab function modelPredictiveControl_v0/Simple Pendulum (Tracking)/r(k) ==
  data: t input; r output
function r = reference_trajectory(t)
    N_x = 30;
    set_point = [5];
    r = kron(ones(N_x, 1), set_point);
end

== matlab function modelPredictiveControl_v0/Pendulum-Cart (Tracking)/MATLAB Function ==
  data: x input; u input; A output; B output; C output; x_k output; y_k output
function [A, B, C, x_k, y_k] = discrete_pendulum_cart_model(x, u)
    coder.extrinsic('ss');
    coder.extrinsic("c2d");
    coder.extrinsic("ssdata");
    % Physical Parameters
    m1 = 1; m2 = 1; ell = 0.1; k = 0; g = 9.81; kappa = 0;

    % Continuous-time model
    Ac = [0 1 0 0;
          k/(m1 + m2 - m2 * cos(x(3))^2) 0 (2*m2*cos(x(3))*ell^2*x(4)^2 + 2*g*m2*cos(2*x(3))*ell + 2*kappa*cos(x(3)) - 2*kappa*x(3)*sin(x(3)))/(ell*(2*m1 + m2 - m2*cos(2*x(3)))) - (4*u*m2*sin(2*x(3)))/(2*m1 + m2 - m2*cos(2*x(3)))^2 - (4*m2*sin(2*x(3))*(kappa*x(3)*cos(x(3)) + ell*k*x(1) + ell^2*m2*x(4)^2*sin(x(3)) + (ell*g*m2*sin(2*x(3)))/2))/(ell*(2*m1 + m2 - m2*cos(2*x(3)))^2) (2*ell*m2*x(4)*sin(x(3)))/(m2*sin(x(3))^2 + m1);
          0 0 0 1;
          -(k*cos(x(3)))/(ell*(- m2*cos(x(3))^2 + m1 + m2)) 0 (ell^2*m2^3*x(4)^2 - kappa*m2^2 - 2*kappa*m1*m2 - kappa*m1^2 + kappa*m2^2*cos(x(3))^2 - ell*g*m2^3*cos(x(3))^3 + ell^2*m1*m2^2*x(4)^2 - ell*u*m2^2*sin(x(3))^3 + kappa*m2^2*x(3)*sin(2*x(3)) + ell*g*m2^3*cos(x(3)) + kappa*m1*m2*cos(x(3))^2 + 2*ell*u*m2^2*sin(x(3)) - ell^2*m2^3*x(4)^2*cos(x(3))^2 - ell*g*m1^2*m2*cos(x(3)) + 2*ell*k*m2^2*x(1)*sin(x(3)) + kappa*m1*m2*x(3)*sin(2*x(3)) - 2*ell^2*m1*m2^2*x(4)^2*cos(x(3))^2 - ell*g*m1*m2^2*cos(x(3))^3 - ell*k*m2^2*x(1)*sin(x(3))^3 + ell*u*m1*m2*sin(x(3)) + ell*k*m1*m2*x(1)*sin(x(3)))/(ell^2*m2*(- m2*cos(x(3))^2 + m1 + m2)^2) -(2*m2*x(4)*sin(2*x(3)))/(2*m1 + m2 - m2*cos(2*x(3)))];
    Bc = [0;
          1/(m1 + m2 - m2 * cos(x(3))^2);
          0;
          (-cos(x(3))/ell) * (1/(m1 + m2 - m2 * cos(x(3))^2))];
    Cc = [1 0 0 0;
          0 0 1 0];
    % Cc = [0 0 1 0];
    Dc = [0; 0];

    % % Discrete-time model Method 1
    % del_t = 0.01;
    % nx = size(Ac, 1);
    % nu = size(Bc, 2);
    % M = expm([[Ac Bc]*del_t; zeros(nu, nx+nu)]);
    % A = M(1:nx, 1:nx);
    % B = M(1:nx, nx+1:nx+nu);
    % C = Cc;
    % D = Dc;

    % Discrete-time model Method 2
    % Preinitializing the sizes of Ad, Bd, Cd, Dd
    A = Ac; B = Bc; C = Cc; D = Dc;
    % Discretization
    del_t = 0.01;
    [A, B, C, D] = ssdata(c2d(ss(Ac,Bc,Cc,Dc),del_t));
    x_k = x;
    y_k = C*x_k;
end
